simulink library "pdc_grc"  (R2024a)
settings: Solver=VariableStepAuto  StartTime=0.0  StopTime=10.0  RelTol=1e-3
undefined symbols (not defined in the file or in its folder): ENUM_IVTROPMODE_ASCHI, ENUM_IVTROPMODE_ASCLO, ENUM_IVTROPMODE_DTCYCTRL, ENUM_IVTROPMODE_FW, ENUM_IVTROPMODE_IVTROFF, KASC_DecDuty_value, KASC_OpenTime_s, KCCM_ASCSwitchEna_flg, KDSM_bIvtrTarHiDebug_flg, KDSM_DiagSpdH_rpm, KDSM_DiagSpdL_rpm, KeMCCR_b_UseMeasCrntDTC, KeSVMR_b_UseStrictClamp, KeSVMR_FullDTCCurr_A, KeSVMR_PWMPrd_cnt, KeSVMR_StrClampMaxDuty_pct, KeSVMR_StrClampMinDuty_pct, KeSVMR_t_DeadTime, KeSVMR_t_MinPulseWidth, KOSP_IvtrTarMor_enum_ovrdflg, KOSP_IvtrTarMor_enum_ovrdval, KPDC_facScalePWM_C, KPDC_FWCnt_C, KPDC_nPosnErrMaxSpd_C, StIvtrMod, StMotMod
libraries: simulink x18, GRC_Lib x6
(part 1 of 3)
settings Model: Creator=FVT22063  LastModifiedBy=FVT22063
settings SFSimCC: SimCustomHeaderCode="#include \"FVTMC_API.h\""  SimUserSources=FVTMC_API.c

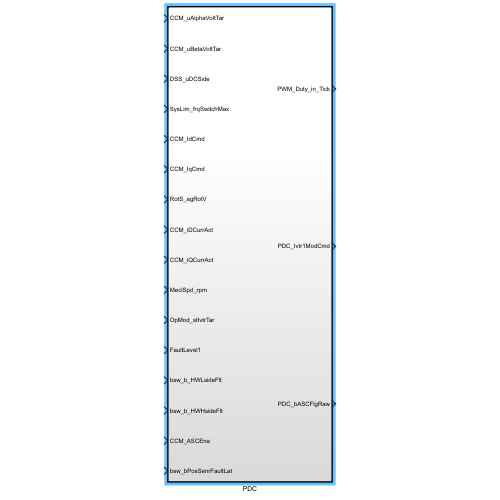
[thumbnail: Simulink's stored preview of the top-level diagram]
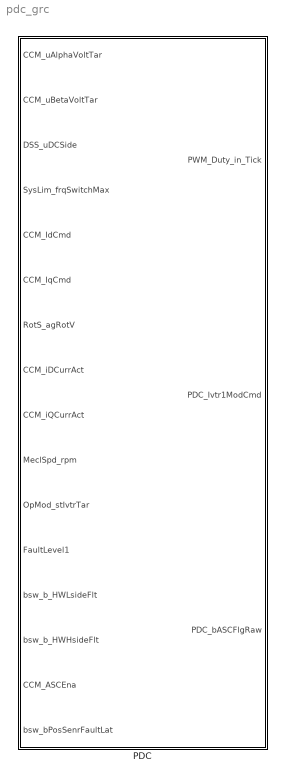
== system pdc_grc ==
  PDC : Subsystem  TreatAsAtomicUnit=on
      settings: RTWSystemCode=Nonreusable function  RTWFcnNameOpts=Use subsystem name  RTWFileNameOpts=Use subsystem name

== system pdc_grc/PDC ==
  CCM_uAlphaVoltTar : Inport  OutDataTypeStr=single
  CCM_uBetaVoltTar : Inport  Port=2  OutDataTypeStr=single
  DSS_uDCSide : Inport  Port=3  OutDataTypeStr=single
  SysLim_frqSwitchMax : Inport  Port=4  OutDataTypeStr=single
  CCM_IdCmd : Inport  Port=5  OutDataTypeStr=single
  CCM_IqCmd : Inport  Port=6  OutDataTypeStr=single
  RotS_agRotV : Inport  Port=7  OutDataTypeStr=single
  CCM_iDCurrAct : Inport  Port=8  OutDataTypeStr=single
  CCM_iQCurrAct : Inport  Port=9  OutDataTypeStr=single
  MeclSpd_rpm : Inport  Port=10  OutDataTypeStr=single
  OpMod_stIvtrTar : Inport  Port=11
  FaultLevel1 : Inport  Port=12  OutDataTypeStr=boolean
  bsw_b_HWLsideFlt : Inport  Port=13  OutDataTypeStr=boolean
  bsw_b_HWHsideFlt : Inport  Port=14  OutDataTypeStr=boolean
  CCM_ASCEna : Inport  Port=15
  bsw_bPosSenrFaultLat : Inport  Port=16  OutDataTypeStr=boolean
  Bus Creator : BusCreator  Inputs=4
  Bus Selector : BusSelector  OutputSignals=CCM_uAlphaVoltTar,CCM_uBetaVoltTar
  Bus Selector1 : BusSelector  OutputSignals=CCM_uAlphaVoltTar,CCM_uBetaVoltTar,DSS_uDCSide,SysLim_frqSwitchMax
  Bus Selector2 : BusSelector  OutputSignals=SysLim_frqSwitchMax
  ChangeTimeCalculation : Subsystem
  PWMCalculation : Subsystem
  SectorDetermine : Subsystem
  WorkTimeCalculation : Subsystem
  PWM_Duty_in_Tick : Outport  VectorParamsAs1DForOutWhenUnconnected=off
  PDC_Ivtr1ModCmd : Outport  Port=2  VectorParamsAs1DForOutWhenUnconnected=off
  PDC_bASCFlgRaw : Outport  Port=3  VectorParamsAs1DForOutWhenUnconnected=off
  wires:
  Bus Creator/1 -> Bus Selector1/1, Bus Selector2/1, Bus Selector/1
  Bus Selector1/1 -> WorkTimeCalculation/1(CCM_uAlphaVoltTar)  "<CCM_uAlphaVoltTar>"
  WorkTimeCalculation/1(PDC_tiWork1) -> ChangeTimeCalculation/1(PDC_tiWork1)
  Bus Selector2/1 -> PWMCalculation/2(SysLim_frqSwitchMax), ChangeTimeCalculation/4(SysLim_frqSwitchMax)  "<SysLim_frqSwitchMax>"
  Bus Selector1/3 -> WorkTimeCalculation/3(DSS_uDCSide)  "<DSS_uDCSide>"
  Bus Selector1/2 -> WorkTimeCalculation/2(CCM_uBetaVoltTar)  "<CCM_uBetaVoltTar>"
  ChangeTimeCalculation/1(PDC_tiChangeAry) -> PWMCalculation/1(PDC_tiChangeAry)
  Bus Selector/2 -> SectorDetermine/2(CCM_uBetaVoltTar)  "<CCM_uBetaVoltTar>"
  SectorDetermine/1(PDC_noSector) -> WorkTimeCalculation/5(PDC_noSector), ChangeTimeCalculation/3(PDC_noSector)
  Bus Selector1/4 -> WorkTimeCalculation/4(SysLim_frqSwitchMax)  "<SysLim_frqSwitchMax>"
  CCM_uAlphaVoltTar/1 -> Bus Creator/2  "CCM_uAlphaVoltTar"
  WorkTimeCalculation/2(PDC_tiWork2) -> ChangeTimeCalculation/2(PDC_tiWork2)
  Bus Selector/1 -> SectorDetermine/1(CCM_uAlphaVoltTar)  "<CCM_uAlphaVoltTar>"
  CCM_uBetaVoltTar/1 -> Bus Creator/3  "CCM_uBetaVoltTar"
  DSS_uDCSide/1 -> Bus Creator/1  "DSS_uDCSide"
  SysLim_frqSwitchMax/1 -> Bus Creator/4  "SysLim_frqSwitchMax"
  PWMCalculation/2(PDC_Ivtr1ModCmd) -> PDC_Ivtr1ModCmd/1
  CCM_IdCmd/1 -> PWMCalculation/3(CCM_IdCmd)
  CCM_IqCmd/1 -> PWMCalculation/4(CCM_IqCmd)
  RotS_agRotV/1 -> PWMCalculation/5(RotS_agRotV)
  CCM_iDCurrAct/1 -> PWMCalculation/6(CCM_iDCurrAct)
  CCM_iQCurrAct/1 -> PWMCalculation/7(CCM_iQCurrAct)
  PWMCalculation/3(PDC_bASCFlgRaw) -> PDC_bASCFlgRaw/1
  OpMod_stIvtrTar/1 -> PWMCalculation/9(OpMod_stIvtrTar)
  MeclSpd_rpm/1 -> PWMCalculation/8(MeclSpd_rpm)
  FaultLevel1/1 -> PWMCalculation/10(FaultLevel2)
  bsw_b_HWLsideFlt/1 -> PWMCalculation/11(bsw_b_HWLsideFlt)
  bsw_b_HWHsideFlt/1 -> PWMCalculation/12(bsw_b_HWHsideFlt)
  CCM_ASCEna/1 -> PWMCalculation/13(CCM_ASCEna)
  bsw_bPosSenrFaultLat/1 -> PWMCalculation/14(bsw_bPosSenrFaultLat)
  PWMCalculation/1(PWM_Duty_in_Tick) -> PWM_Duty_in_Tick/1

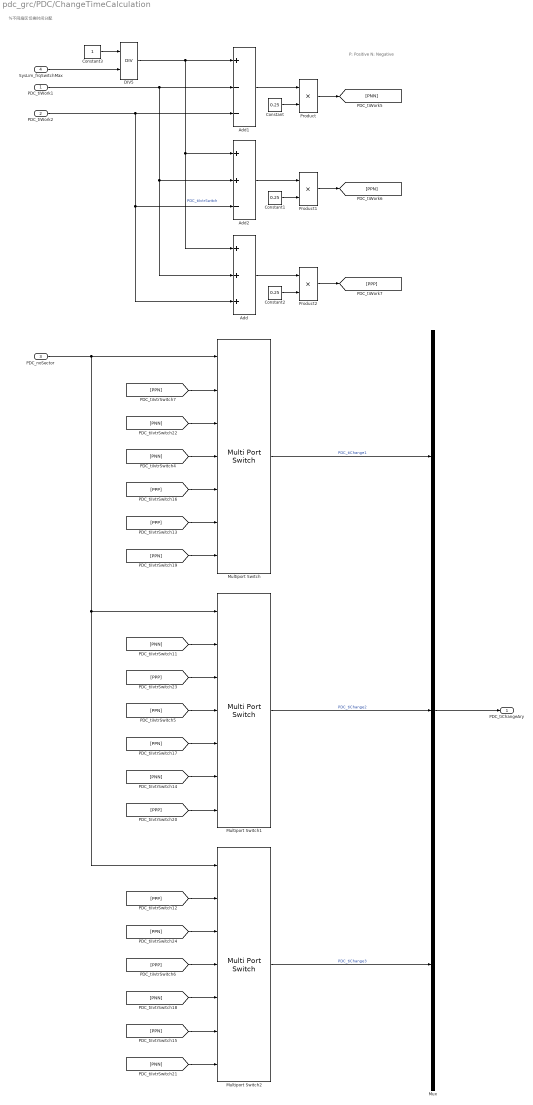
== system pdc_grc/PDC/ChangeTimeCalculation ==
  note: P: Positive
      | N: Negative
  note: %不同扇区切换时间分配
  PDC_tiWork1 : Inport  OutDataTypeStr=single
  PDC_tiWork2 : Inport  Port=2  OutDataTypeStr=single
  PDC_noSector : Inport  Port=3  OutDataTypeStr=single
  SysLim_frqSwitchMax : Inport  Port=4  OutDataTypeStr=single
  Add : Sum  Inputs=+++
  Add1 : Sum  Inputs=+--
  Add2 : Sum  Inputs=++-
  Constant : Constant  Value=0.25  OutDataTypeStr=single
  Constant1 : Constant  Value=0.25  OutDataTypeStr=single
  Constant2 : Constant  Value=0.25  OutDataTypeStr=single
  Constant3 : Constant  OutDataTypeStr=single
  DIV5 : GRC_Lib/ArithmeticOperations/DIV  MinDivVal=1e-15  IpDT=single
  Multiport Switch : MultiPortSwitch  Inputs=6  DiagnosticForDefault=None  SaturateOnIntegerOverflow=off  InputSameDT=off
  Multiport Switch1 : MultiPortSwitch  Inputs=6  DiagnosticForDefault=None  SaturateOnIntegerOverflow=off  InputSameDT=off
  Multiport Switch2 : MultiPortSwitch  Inputs=6  DiagnosticForDefault=None  SaturateOnIntegerOverflow=off  InputSameDT=off
  Mux : Mux  Inputs=3
  Product : Product
  Product1 : Product
  Product2 : Product
  PDC_tiChangeAry : Outport  OutDataTypeStr=single  VectorParamsAs1DForOutWhenUnconnected=off
  wires:
  DIV5/1 -> Add/1, Add2/1, Add1/1  "PDC_tiIvtrSwitch"
  PDC_tiWork1/1 -> Add/2, Add2/2, Add1/2
  PDC_tiWork2/1 -> Add1/3, Add/3, Add2/3
  PDC_noSector/1 -> Multiport Switch2/1, Multiport Switch1/1, Multiport Switch/1
  Add1/1 -> Product/1
  Product/1 -> [PNN]
  Constant/1 -> Product/2
  Constant1/1 -> Product1/2
  Product1/1 -> [PPN]
  Add2/1 -> Product1/1
  Add/1 -> Product2/1
  Product2/1 -> [PPP]
  Constant2/1 -> Product2/2
  Multiport Switch/1 -> Mux/1  "PDC_tiChange1"
  Multiport Switch1/1 -> Mux/2  "PDC_tiChange2"
  Multiport Switch2/1 -> Mux/3  "PDC_tiChange3"
  [PNN] -> Multiport Switch/4
  [PPN] -> Multiport Switch1/4
  [PPP] -> Multiport Switch2/4
  [PPN] -> Multiport Switch/2
  [PNN] -> Multiport Switch1/2
  [PPP] -> Multiport Switch2/2
  [PPP] -> Multiport Switch/6
  [PNN] -> Multiport Switch1/6
  [PPN] -> Multiport Switch2/6
  [PPP] -> Multiport Switch/5
  [PPN] -> Multiport Switch1/5
  [PNN] -> Multiport Switch2/5
  [PPN] -> Multiport Switch/7
  [PPP] -> Multiport Switch1/7
  [PNN] -> Multiport Switch2/7
  [PNN] -> Multiport Switch/3
  [PPP] -> Multiport Switch1/3
  [PPN] -> Multiport Switch2/3
  SysLim_frqSwitchMax/1 -> DIV5/2
  Constant3/1 -> DIV5/1
  Mux/1 -> PDC_tiChangeAry/1

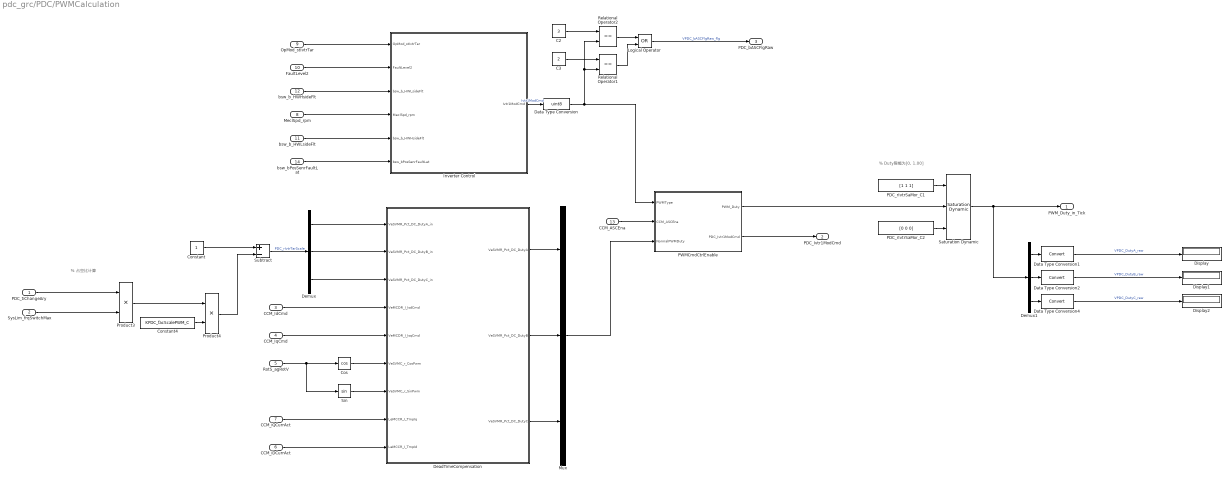
== system pdc_grc/PDC/PWMCalculation ==
  note: % 占空比计算
  note: % Duty限幅为[0, 1.00]
  PDC_tiChangeAry : Inport
  SysLim_frqSwitchMax : Inport  Port=2  OutDataTypeStr=single
  CCM_IdCmd : Inport  Port=3  OutDataTypeStr=single
  CCM_IqCmd : Inport  Port=4  OutDataTypeStr=single
  RotS_agRotV : Inport  Port=5  OutDataTypeStr=single
  CCM_iDCurrAct : Inport  Port=6  OutDataTypeStr=single
  CCM_iQCurrAct : Inport  Port=7  OutDataTypeStr=single
  MeclSpd_rpm : Inport  Port=8  OutDataTypeStr=single
  OpMod_stIvtrTar : Inport  Port=9
  FaultLevel2 : Inport  Port=10  OutDataTypeStr=boolean
  bsw_b_HWLsideFlt : Inport  Port=11
  bsw_b_HWHsideFlt : Inport  Port=12
  CCM_ASCEna : Inport  Port=13
  bsw_bPosSenrFaultLat : Inport  Port=14  OutDataTypeStr=boolean
  C2 : Constant  Value=3  OutDataTypeStr=uint8  SampleTime=-1
  C3 : Constant  Value=2  OutDataTypeStr=uint8  SampleTime=-1
  Constant : Constant  OutDataTypeStr=Inherit: Inherit via back propagation
  Constant4 : Constant  Value=KPDC_facScalePWM_C
  Cos : Trigonometry  Operator=cos
  Data Type Conversion : DataTypeConversion  OutDataTypeStr=uint8  SaturateOnIntegerOverflow=off  RndMeth=Floor
  Data Type Conversion1 : DataTypeConversion  SaturateOnIntegerOverflow=off  RndMeth=Floor
  Data Type Conversion2 : DataTypeConversion  SaturateOnIntegerOverflow=off  RndMeth=Floor
  Data Type Conversion4 : DataTypeConversion  SaturateOnIntegerOverflow=off  RndMeth=Floor
  DeadTimeCompensation : Subsystem
  Demux : Demux  Outputs=3
  Demux1 : Demux  Outputs=3
  Display : Display
  Display1 : Display
  Display2 : Display
  "Inverter Control " : Subsystem
  Logical Operator : Logic  Operator=OR  AllPortsSameDT=off  OutDataTypeStr=boolean
  Mux : Mux  Inputs=3
  PDC_rIvtrSaMor_C1 : Constant  Value=[1 1 1]
  PDC_rIvtrSaMor_C2 : Constant  Value=[0 0 0]
  PWMCmdCtrlEnable : Subsystem
      settings: FunctionInterfaceSpec=Allow arguments (Optimized)
  Product3 : Product
  Product4 : Product
  Relational Operator1 : RelationalOperator  Operator===  OutDataTypeStr=boolean  RndMeth=Simplest  InputSameDT=off
  Relational Operator2 : RelationalOperator  Operator===  OutDataTypeStr=boolean  RndMeth=Simplest  InputSameDT=off
  Saturation Dynamic : simulink/Discontinuities/Saturation Dynamic  OutMin=[]  OutMax=[]  OutDataTypeStr=Inherit: Same as second input  OutDataType=fixdt(1, 16)  OutScaling=2^-10  DoSatur=off
  Sin : Trigonometry
  Subtract : Sum  Inputs=+-
  PWM_Duty_in_Tick : Outport
  PDC_Ivtr1ModCmd : Outport  Port=2  OutDataTypeStr=uint8  VectorParamsAs1DForOutWhenUnconnected=off
  PDC_bASCFlgRaw : Outport  Port=3  VectorParamsAs1DForOutWhenUnconnected=off
  wires:
  Product4/1 -> Subtract/2
  PDC_rIvtrSaMor_C2/1 -> Saturation Dynamic/3
  PDC_rIvtrSaMor_C1/1 -> Saturation Dynamic/1
  Constant4/1 -> Product4/2
  Product3/1 -> Product4/1
  SysLim_frqSwitchMax/1 -> Product3/2
  PDC_tiChangeAry/1 -> Product3/1
  Saturation Dynamic/1 -> Demux1/1, PWM_Duty_in_Tick/1
  Cos/1 -> DeadTimeCompensation/6(VeSVMC_r_CosPwm)
  CCM_IdCmd/1 -> DeadTimeCompensation/4(VeMCDR_I_IsdCmd)
  Demux/1 -> DeadTimeCompensation/1(VeSVMR_Pct_DC_DutyA_in)
  Sin/1 -> DeadTimeCompensation/7(VeSVMC_r_SinPwm)
  Demux/2 -> DeadTimeCompensation/2(VeSVMR_Pct_DC_DutyB_in)
  CCM_IqCmd/1 -> DeadTimeCompensation/5(VeMCDR_I_IsqCmd)
  Demux/3 -> DeadTimeCompensation/3(VeSVMR_Pct_DC_DutyC_in)
  RotS_agRotV/1 -> Sin/1, Cos/1
  DeadTimeCompensation/1(VeSVMR_Pct_DC_DutyA) -> Mux/1
  DeadTimeCompensation/2(VeSVMR_Pct_DC_DutyB) -> Mux/2
  DeadTimeCompensation/3(VeSVMR_Pct_DC_DutyC) -> Mux/3
  PWMCmdCtrlEnable/1(PWM_Duty) -> Saturation Dynamic/2
  Constant/1 -> Subtract/1
  Subtract/1 -> Demux/1  "PDC_rIvtrTarScale"
  PWMCmdCtrlEnable/2(PDC_Ivtr1ModCmd) -> PDC_Ivtr1ModCmd/1
  Mux/1 -> PWMCmdCtrlEnable/3(NormalPWMDuty)
  CCM_iQCurrAct/1 -> DeadTimeCompensation/8(LeMCCR_I_TmpIq)
  CCM_iDCurrAct/1 -> DeadTimeCompensation/9(LeMCCR_I_TmpId)
  OpMod_stIvtrTar/1 -> "Inverter Control "/1(OpMod_stIvtrTar)
  MeclSpd_rpm/1 -> "Inverter Control "/4(MeclSpd_rpm)
  "Inverter Control "/1(Ivtr1ModCmd) -> Data Type Conversion/1  "Ivtr1ModCmd"
  bsw_b_HWLsideFlt/1 -> "Inverter Control "/5(bsw_b_HWHsideFlt)
  FaultLevel2/1 -> "Inverter Control "/2(FaultLevel2)
  bsw_b_HWHsideFlt/1 -> "Inverter Control "/3(bsw_b_HWLsideFlt)
  Data Type Conversion/1 -> Relational Operator2/2, Relational Operator1/2, PWMCmdCtrlEnable/1(PWMType)
  CCM_ASCEna/1 -> PWMCmdCtrlEnable/2(CCM_ASCEna)
  C2/1 -> Relational Operator2/1
  C3/1 -> Relational Operator1/1
  Relational Operator2/1 -> Logical Operator/1
  Relational Operator1/1 -> Logical Operator/2
  Logical Operator/1 -> PDC_bASCFlgRaw/1  "VPDC_bASCFlgRaw_flg"
  bsw_bPosSenrFaultLat/1 -> "Inverter Control "/6(bsw_bPosSenrFaultLat)
  Demux1/1 -> Data Type Conversion1/1
  Demux1/2 -> Data Type Conversion2/1
  Demux1/3 -> Data Type Conversion4/1
  Data Type Conversion1/1 -> Display/1  "VPDC_DutyA_raw"
  Data Type Conversion2/1 -> Display1/1  "VPDC_DutyB_raw"
  Data Type Conversion4/1 -> Display2/1  "VPDC_DutyC_raw"

== system pdc_grc/PDC/SectorDetermine ==
  note: 扇区
      | Ⅰ
      | Ⅱ
      | Ⅲ
      | Ⅳ
      | Ⅴ
      | Ⅵ
      |
      | N
      | 3
      | 1
      | 5
      | 4
      | 6
      | 2
  note: C
  note: B
  note: A
  note: %扇区判断
  CCM_uAlphaVoltTar : Inport  OutDataTypeStr=single
  CCM_uBetaVoltTar : Inport  Port=2  OutDataTypeStr=single
  Add : Sum  Inputs=3
  Constant : Constant  Value=0.866  OutDataTypeStr=single
  Constant1 : Constant  Value=0.5  OutDataTypeStr=single
  Constant2 : Constant  Value=-1  OutDataTypeStr=single
  Constant3 : Constant  Value=0  OutDataTypeStr=single
  Constant4 : Constant  Value=2  OutDataTypeStr=single
  Constant5 : Constant  Value=4  OutDataTypeStr=single
  Constant6 : Constant  OutDataTypeStr=single
  Product{,1..5} (6 alike) : Product
  Relational Operator : RelationalOperator  OutDataTypeStr=boolean  RndMeth=Simplest  InputSameDT=off
  Relational Operator1 : RelationalOperator  OutDataTypeStr=boolean  RndMeth=Simplest  InputSameDT=off
  Relational Operator2 : RelationalOperator  OutDataTypeStr=boolean  RndMeth=Simplest  InputSameDT=off
  PDC_noSector : Outport  OutDataTypeStr=single  VectorParamsAs1DForOutWhenUnconnected=off
  wires:
  CCM_uAlphaVoltTar/1 -> Product/1  "CCM_uAlphaVoltTar"
  Constant/1 -> Product/2
  CCM_uBetaVoltTar/1 -> Relational Operator2/1, Product1/1  "CCM_uBetaVoltTar"
  Constant1/1 -> Product1/2
  Product/1 -> Product2/1, Relational Operator/1
  Product1/1 -> Relational Operator/2, Relational Operator1/2
  Product2/1 -> Relational Operator1/1
  Constant2/1 -> Product2/2
  Constant3/1 -> Relational Operator2/2
  Relational Operator/1 -> Product3/1
  Constant4/1 -> Product3/2
  Constant5/1 -> Product4/2
  Relational Operator1/1 -> Product4/1
  Constant6/1 -> Product5/2
  Relational Operator2/1 -> Product5/1
  Product3/1 -> Add/1
  Product4/1 -> Add/2
  Product5/1 -> Add/3
  Add/1 -> PDC_noSector/1  "PDC_noSector"

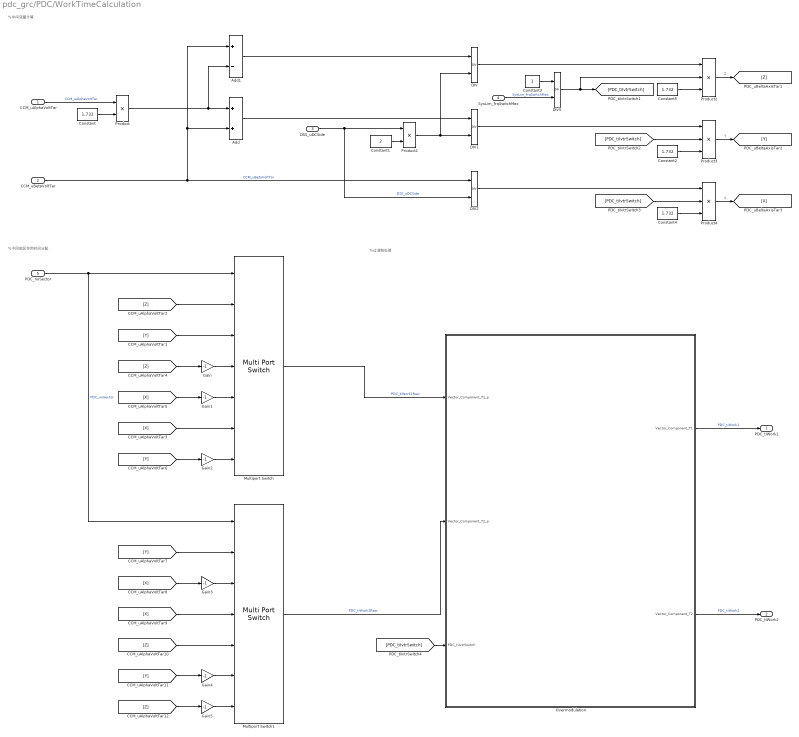
== system pdc_grc/PDC/WorkTimeCalculation ==
  note: %过调制处理
  note: %中间变量计算
  note: %不同扇区作用时间分配
  CCM_uAlphaVoltTar : Inport  OutDataTypeStr=single
  CCM_uBetaVoltTar : Inport  Port=2  OutDataTypeStr=single
  DSS_uDCSide : Inport  Port=3  OutDataTypeStr=single
  SysLim_frqSwitchMax : Inport  Port=4  OutDataTypeStr=single
  PDC_noSector : Inport  Port=5  OutDataTypeStr=single
  Add : Sum
  Add1 : Sum  Inputs=+-
  Constant{,2,4..5} (4 alike) : Constant  Value=1.732  OutDataTypeStr=single
  Constant1 : Constant  Value=2  OutDataTypeStr=single
  Constant3 : Constant  OutDataTypeStr=single
  DIV{,1..2,5} (4 alike) : GRC_Lib/ArithmeticOperations/DIV  MinDivVal=1e-15  IpDT=single
  Gain{,1..5} (6 alike) : Gain  Gain=-1
  Multiport Switch : MultiPortSwitch  Inputs=6  DiagnosticForDefault=None  SaturateOnIntegerOverflow=off  InputSameDT=off
  Multiport Switch1 : MultiPortSwitch  Inputs=6  DiagnosticForDefault=None  SaturateOnIntegerOverflow=off  InputSameDT=off
  Overmodulation : Subsystem
  Product : Product
  Product1 : Product
  Product2 : Product  Inputs=3
  Product3 : Product  Inputs=3
  Product4 : Product  Inputs=3
  PDC_tiWork1 : Outport  OutDataTypeStr=single  VectorParamsAs1DForOutWhenUnconnected=off
  PDC_tiWork2 : Outport  Port=2  OutDataTypeStr=single  VectorParamsAs1DForOutWhenUnconnected=off
  wires:
  Constant/1 -> Product/2
  CCM_uAlphaVoltTar/1 -> Product/1  "CCM_uAlphaVoltTar"
  Product/1 -> Add1/2, Add/1
  Add1/1 -> DIV/1
  Constant1/1 -> Product1/2
  DIV/1 -> Product2/1
  Constant5/1 -> Product2/3
  DIV5/1 -> [PDC_tiIvtrSwitch], Product2/2
  Product2/1 -> [Z]  "Z"
  Product3/1 -> [Y]  "Y"
  Constant2/1 -> Product3/3
  DIV1/1 -> Product3/1
  Product1/1 -> DIV/2, DIV1/2
  DSS_uDCSide/1 -> DIV2/2, Product1/1  "DSS_uDCSide"
  Add/1 -> DIV1/1
  CCM_uBetaVoltTar/1 -> Add1/1, Add/2, DIV2/1  "CCM_uBetaVoltTar"
  DIV2/1 -> Product4/1
  Constant4/1 -> Product4/3
  Product4/1 -> [X]  "X"
  PDC_noSector/1 -> Multiport Switch1/1, Multiport Switch/1  "PDC_noSector"
  [Z] -> Multiport Switch/2
  [Y] -> Multiport Switch/3
  [Z] -> Gain/1
  Gain/1 -> Multiport Switch/4
  [X] -> Multiport Switch/6
  [X] -> Gain1/1
  Gain1/1 -> Multiport Switch/5
  [Y] -> Gain2/1
  Gain2/1 -> Multiport Switch/7
  [Y] -> Multiport Switch1/2
  Gain3/1 -> Multiport Switch1/3
  [X] -> Gain3/1
  [X] -> Multiport Switch1/4
  [Z] -> Multiport Switch1/5
  Gain4/1 -> Multiport Switch1/6
  [Y] -> Gain4/1
  Gain5/1 -> Multiport Switch1/7
  [Z] -> Gain5/1
  Overmodulation/1(Vector_Component_T1) -> PDC_tiWork1/1  "PDC_tiWork1"
  Overmodulation/2(Vector_Component_T2) -> PDC_tiWork2/1  "PDC_tiWork2"
  [PDC_tiIvtrSwitch] -> Product3/2
  [PDC_tiIvtrSwitch] -> Product4/2
  SysLim_frqSwitchMax/1 -> DIV5/2  "SysLim_frqSwitchMax"
  Constant3/1 -> DIV5/1
  Multiport Switch/1 -> Overmodulation/1(Vector_Component_T1_p)  "PDC_tiWork1Raw"
  Multiport Switch1/1 -> Overmodulation/2(Vector_Component_T2_p)  "PDC_tiWork2Raw"
  [PDC_tiIvtrSwitch] -> Overmodulation/3(PDC_tiIvtrSwitch)

== system pdc_grc/PDC/PWMCalculation/DeadTimeCompensation ==
  VeSVMR_Pct_DC_DutyA_in : Inport
  VeSVMR_Pct_DC_DutyB_in : Inport  Port=2
  VeSVMR_Pct_DC_DutyC_in : Inport  Port=3
  VeMCDR_I_IsdCmd : Inport  Port=4
  VeMCDR_I_IsqCmd : Inport  Port=5
  VeSVMC_r_CosPwm : Inport  Port=6
  VeSVMC_r_SinPwm : Inport  Port=7
  LeMCCR_I_TmpIq : Inport  Port=8
  LeMCCR_I_TmpId : Inport  Port=9
  MngSVMR_Base_MtrCntrl0_ProcessDCsForHWIO : Subsystem  RTWFcnName=MngSVMR_Base_MtrCntrl0_ProcessDCsForHWIO  RTWFileName=svmcmbas
      settings: RTWSystemCode=Nonreusable function  RTWFcnNameOpts=User specified  RTWFileNameOpts=User specified
  ReInitSVMR_DeadTimeCompensation : Subsystem  TreatAsAtomicUnit=on  RTWFcnName=ReInitSVMR_DeadTimeCompensation  RTWFileName=svmcmbas
      settings: RTWFcnNameOpts=User specified  RTWFileNameOpts=User specified
  ReInitSVMR_PWM_Modulation : Subsystem  TreatAsAtomicUnit=on  RTWFcnName=ReInitSVMR_PWM_Modulation  RTWFileName=svmcmbas
      settings: RTWFcnNameOpts=User specified  RTWFileNameOpts=User specified
  ReciSqrt3M1 : Constant  Value=KeMCCR_b_UseMeasCrntDTC  OutDataTypeStr=uint8
      settings: AttributesFormatString=dd_value = 0
  ReciSqrt3M2 : Constant  OutDataTypeStr=uint8
      settings: AttributesFormatString=dd_value = 1
  ReciSqrt3M3 : Constant  OutDataTypeStr=uint8
      settings: AttributesFormatString=dd_value = 1
  Terminator : Terminator
  Terminator1 : Terminator
  Terminator2 : Terminator
  VeSVMR_Pct_DC_DutyA : Outport  VectorParamsAs1DForOutWhenUnconnected=off
  VeSVMR_Pct_DC_DutyB : Outport  Port=2  VectorParamsAs1DForOutWhenUnconnected=off
  VeSVMR_Pct_DC_DutyC : Outport  Port=3  VectorParamsAs1DForOutWhenUnconnected=off
  wires:
  MngSVMR_Base_MtrCntrl0_ProcessDCsForHWIO/4(VeSVMR_Pct_DC_DutyA) -> VeSVMR_Pct_DC_DutyA/1
  MngSVMR_Base_MtrCntrl0_ProcessDCsForHWIO/5(VeSVMR_Pct_DC_DutyB) -> VeSVMR_Pct_DC_DutyB/1
  VeSVMR_Pct_DC_DutyB_in/1 -> MngSVMR_Base_MtrCntrl0_ProcessDCsForHWIO/3(VeSVMR_Pct_DC_DutyB_in)
  MngSVMR_Base_MtrCntrl0_ProcessDCsForHWIO/1(VeSVMR_Pct_DC_DutyA_Cmd) -> Terminator/1
  MngSVMR_Base_MtrCntrl0_ProcessDCsForHWIO/6(VeSVMR_Pct_DC_DutyC) -> VeSVMR_Pct_DC_DutyC/1
  MngSVMR_Base_MtrCntrl0_ProcessDCsForHWIO/2(VeSVMR_Pct_DC_DutyB_Cmd) -> Terminator1/1
  VeSVMR_Pct_DC_DutyA_in/1 -> MngSVMR_Base_MtrCntrl0_ProcessDCsForHWIO/2(VeSVMR_Pct_DC_DutyA_in)
  ReciSqrt3M3/1 -> MngSVMR_Base_MtrCntrl0_ProcessDCsForHWIO/1(VeGDCR_e_EffectivePwrStageCmd)
  MngSVMR_Base_MtrCntrl0_ProcessDCsForHWIO/3(VeSVMR_Pct_DC_DutyC_Cmd) -> Terminator2/1
  VeMCDR_I_IsqCmd/1 -> MngSVMR_Base_MtrCntrl0_ProcessDCsForHWIO/6(VeMCDR_I_IsqCmd)
  VeSVMR_Pct_DC_DutyC_in/1 -> MngSVMR_Base_MtrCntrl0_ProcessDCsForHWIO/4(VeSVMR_Pct_DC_DutyC_in)
  VeMCDR_I_IsdCmd/1 -> MngSVMR_Base_MtrCntrl0_ProcessDCsForHWIO/5(VeMCDR_I_IsdCmd)
  VeSVMC_r_CosPwm/1 -> MngSVMR_Base_MtrCntrl0_ProcessDCsForHWIO/7(VeSVMC_r_CosPwm)
  VeSVMC_r_SinPwm/1 -> MngSVMR_Base_MtrCntrl0_ProcessDCsForHWIO/8(VeSVMC_r_SinPwm)
  LeMCCR_I_TmpIq/1 -> MngSVMR_Base_MtrCntrl0_ProcessDCsForHWIO/18(LeMCCR_I_TmpIq)
  LeMCCR_I_TmpId/1 -> MngSVMR_Base_MtrCntrl0_ProcessDCsForHWIO/19(LeMCCR_I_TmpId)
  ReciSqrt3M2/1 -> MngSVMR_Base_MtrCntrl0_ProcessDCsForHWIO/11(VeSVMR_e_PWM_Type)
  ReInitSVMR_DeadTimeCompensation/1(VeSVMR_K_DeadTimeCmp_Slope) -> MngSVMR_Base_MtrCntrl0_ProcessDCsForHWIO/9(VaSVMR_K_DeadTimeCmp_Slope)
  ReInitSVMR_DeadTimeCompensation/2(VeSVMR_Pct_DeadTimeCmp) -> MngSVMR_Base_MtrCntrl0_ProcessDCsForHWIO/10(VaSVMR_Pct_DeadTimeCmp)
  ReInitSVMR_PWM_Modulation/1(VeSVMR_Pct_DC_FixedDutyOffset) -> MngSVMR_Base_MtrCntrl0_ProcessDCsForHWIO/12(VeSVMR_Pct_DC_FixedDutyOffset)
  ReInitSVMR_PWM_Modulation/2(VeSVMR_Pct_DCMaxDuty_nom) -> MngSVMR_Base_MtrCntrl0_ProcessDCsForHWIO/13(VaSVMR_Pct_DCMaxDuty_nom)
  ReInitSVMR_PWM_Modulation/3(VeSVMR_Pct_DCMinDuty_nom) -> MngSVMR_Base_MtrCntrl0_ProcessDCsForHWIO/14(VaSVMR_Pct_DCMinDuty_nom)
  ReInitSVMR_PWM_Modulation/4(VeSVMR_Pct_DCMaxDutyRound) -> MngSVMR_Base_MtrCntrl0_ProcessDCsForHWIO/15(VaSVMR_Pct_DCMaxDutyRound)
  ReInitSVMR_PWM_Modulation/5(VeSVMR_Pct_DCMinDutyRound) -> MngSVMR_Base_MtrCntrl0_ProcessDCsForHWIO/16(VaSVMR_Pct_DCMinDutyRound)
  ReciSqrt3M1/1 -> MngSVMR_Base_MtrCntrl0_ProcessDCsForHWIO/17(VeMCCR_b_UseMeasCrntDTC)

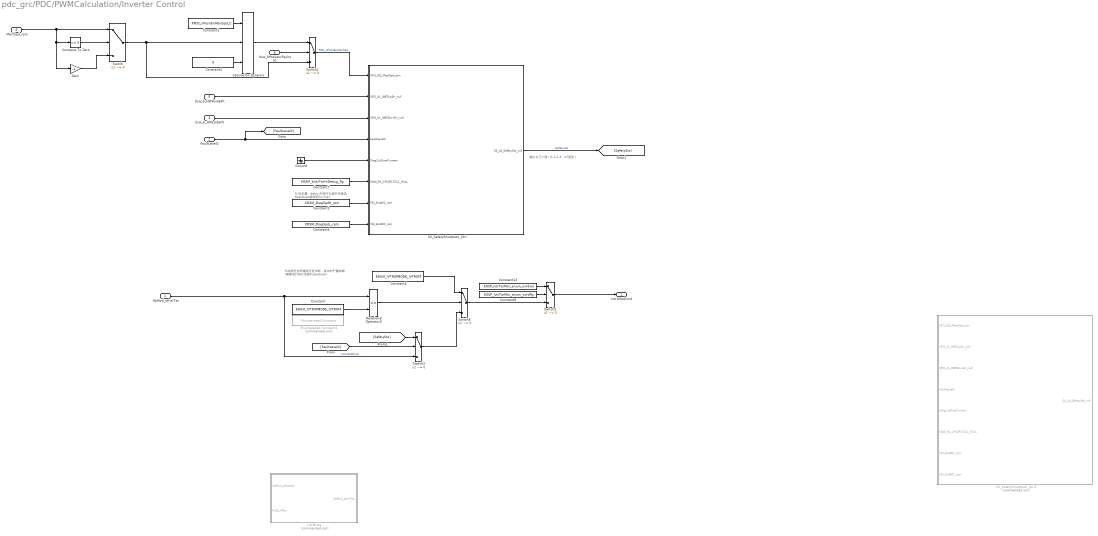
== system pdc_grc/PDC/PWMCalculation/Inverter Control  ==
  note: % 标定量，debug时候可以使开关管由
      | freewheel跳转到normal
  note: 输出为几个值（0-1-2-3，u8类型）
  note: %快速任务和慢速任务诊断，其中的严重故障
      | (需要进行ASC或者Freewheel)
  OpMod_stIvtrTar : Inport
  FaultLevel2 : Inport  Port=2  OutDataTypeStr=boolean
  bsw_b_HWLsideFlt : Inport  Port=3
  MeclSpd_rpm : Inport  Port=4  OutDataTypeStr=single
  bsw_b_HWHsideFlt : Inport  Port=5
  bsw_bPosSenrFaultLat : Inport  Port=6  OutDataTypeStr=boolean
  Compare To Zero : simulink/Logic and Bit Operations/Compare To Zero  relop=>=  OutDataTypeStr=boolean
  Constant : Constant  Value=ENUM_IVTROPMODE_IVTROFF
  Constant1 : Constant  Value=KPDC_nPosnErrMaxSpd_C
  Constant12 : Constant  Value=KOSP_IvtrTarMor_enum_ovrdval  SampleTime=-1
  Constant2 : Constant  Value=KDSM_DiagSpdH_rpm  SampleTime=-1
  Constant3 : Constant  Value=0  OutDataTypeStr=single
  Constant4 : Constant  Value=KDSM_DiagSpdL_rpm  SampleTime=-1
  Constant5 : Constant  Value=ENUM_IVTROPMODE_IVTROFF
  Constant7 : Constant  Value=KDSM_bIvtrTarHiDebug_flg  OutDataTypeStr=boolean  SampleTime=-1
  Constant9 : Constant  Value=KOSP_IvtrTarMor_enum_ovrdflg  OutDataTypeStr=boolean  SampleTime=-1
  Enumerated Constant1 : simulink/Sources/Enumerated Constant  Commented=on  OutDataTypeStr=Enum: StIvtrMod  Value=StIvtrMod.StIvtrModIvtrOffMod  SampleTime=inf
  Gain : Gain  Gain=-1  OutDataTypeStr=single
  Ground : Ground
  IvtrMode : Subsystem  Commented=on
  Relational Operator2 : RelationalOperator  Operator===  OutDataTypeStr=boolean  RndMeth=Simplest  InputSameDT=off
  SS_SafetyShutdown_Ctrl : Stateflow chart  TreatAsAtomicUnit=on
  SS_SafetyShutdown_Ctrl1 : Stateflow chart  Commented=on  TreatAsAtomicUnit=on
  Saturation Dynamic : simulink/Discontinuities/Saturation Dynamic  OutMin=[]  OutMax=[]  OutDataTypeStr=Inherit: Same as second input  OutDataType=fixdt(1, 16)  OutScaling=2^-10  DoSatur=off
  Switch{,1..3,5} (5 alike) : Switch  Criteria=u2 ~= 0  SaturateOnIntegerOverflow=off  InputSameDT=off
  Ivtr1ModCmd : Outport
  wires:
  Switch5/1 -> Switch2/3
  bsw_b_HWLsideFlt/1 -> SS_SafetyShutdown_Ctrl/3(SPI2_b1_IGBTDwnErr_null)
  FaultLevel2/1 -> [FaultLevel2], SS_SafetyShutdown_Ctrl/4(FaultLevel2)
  Constant12/1 -> Switch2/1
  Switch2/1 -> Ivtr1ModCmd/1
  Constant9/1 -> Switch2/2
  Gain/1 -> Switch/3
  Constant7/1 -> SS_SafetyShutdown_Ctrl/6(DIAG_B1_CPLDFLTCLC_NULL)
  MeclSpd_rpm/1 -> Switch/1, Compare To Zero/1, Gain/1
  Compare To Zero/1 -> Switch/2
  SS_SafetyShutdown_Ctrl/1(SS_u8_SafetySts_null) -> [SafetySts]  "SafetySts"
  bsw_b_HWHsideFlt/1 -> SS_SafetyShutdown_Ctrl/2(SPI2_b1_IGBTUpErr_null)
  Ground/1 -> SS_SafetyShutdown_Ctrl/5(Diag1_bOverCurrent)
  Constant/1 -> Relational Operator2/2
  Relational Operator2/1 -> Switch5/2
  Constant5/1 -> Switch5/1
  Switch3/1 -> Switch5/3
  [FaultLevel2] -> Switch3/2
  [SafetySts] -> Switch3/1
  Constant4/1 -> SS_SafetyShutdown_Ctrl/8(f32_ExtASC_rpm)
  Constant2/1 -> SS_SafetyShutdown_Ctrl/7(f32_EntASC_rpm)
  OpMod_stIvtrTar/1 -> Relational Operator2/1, Switch3/3  "Ivtr1ModCmd"
  Constant1/1 -> Saturation Dynamic/1
  Saturation Dynamic/1 -> Switch1/1
  Switch/1 -> Switch1/3, Saturation Dynamic/2
  Constant3/1 -> Saturation Dynamic/3
  bsw_bPosSenrFaultLat/1 -> Switch1/2
  Switch1/1 -> SS_SafetyShutdown_Ctrl/1(SPI1_f32_MeclSpd_rpm)  "PDC_nPosnErrMaxSpd"

== system pdc_grc/PDC/PWMCalculation/PWMCmdCtrlEnable ==
  PWMType : Inport
  CCM_ASCEna : Inport  Port=2
  NormalPWMDuty : Inport  Port=3
  C1 : Constant  OutDataTypeStr=uint8  SampleTime=-1
  C2 : Constant  Value=2  OutDataTypeStr=uint8  SampleTime=-1
  C3 : Constant  Value=3  OutDataTypeStr=uint8  SampleTime=-1
  C4 : Constant  Value=0  OutDataTypeStr=uint8  SampleTime=-1
  If : If  NumInputs=5  IfExpression=u1==u2  ElseIfExpressions=(u1==u3|u1==u4),u1==u5
  Merge : Merge  Inputs=4
  Merge2 : Merge  Inputs=4
  NormalPWM : Subsystem  TreatAsAtomicUnit=on
      settings: RTWFcnNameOpts=Use subsystem name
  PWMFW : Subsystem  TreatAsAtomicUnit=on
      settings: RTWFcnNameOpts=Use subsystem name
  PWMGOFF : Subsystem  TreatAsAtomicUnit=on
      settings: RTWFcnNameOpts=Use subsystem name
  ThreePhaseSC : Subsystem  TreatAsAtomicUnit=on
      settings: RTWFcnNameOpts=Use subsystem name
  ThreePhaseSC1 : Subsystem  Commented=on  TreatAsAtomicUnit=on
      settings: RTWFcnNameOpts=Use subsystem name
  PWM_Duty : Outport  VectorParamsAs1DForOutWhenUnconnected=off
  PDC_Ivtr1ModCmd : Outport  Port=2  VectorParamsAs1DForOutWhenUnconnected=off
  wires:
  If/1 -> NormalPWM/Action
  NormalPWM/1(PWM_Duty) -> Merge/1
  Merge/1 -> PWM_Duty/1
  If/3 -> PWMFW/Action
  PWMType/1 -> [PWMType], If/1
  C1/1 -> If/2
  If/2 -> ThreePhaseSC/Action
  ThreePhaseSC/1(PWM_Duty) -> Merge/2
  PWMFW/1(PWM_Duty) -> Merge/3
  NormalPWM/2(PDC_Ivtr1ModCmd) -> Merge2/1
  ThreePhaseSC/2(PDC_Ivtr1ModCmd) -> Merge2/2
  PWMFW/2(PDC_Ivtr1ModCmd) -> Merge2/3
  C4/1 -> If/5
  [PWMType] -> ThreePhaseSC/2(PWMType)
  If/4 -> PWMGOFF/Action
  [PWMType] -> PWMGOFF/1(PWMType)
  PWMGOFF/1(PWM_Duty) -> Merge/4
  PWMGOFF/2(PDC_Ivtr1ModCmd) -> Merge2/4
  NormalPWMDuty/1 -> ThreePhaseSC/1(NormalPWMDuty), NormalPWM/1(Normal_PWM_Duty)
  C2/1 -> If/3
  C3/1 -> If/4
  CCM_ASCEna/1 -> ThreePhaseSC/3(CCM_ASCEna)
  Merge2/1 -> PDC_Ivtr1ModCmd/1  "VPDC_Ivtr1ModCmd_enum"

== system pdc_grc/PDC/WorkTimeCalculation/Overmodulation ==
  Vector_Component_T1_p : Inport  OutDataTypeStr=single
  Vector_Component_T2_p : Inport  Port=2  OutDataTypeStr=single
  PDC_tiIvtrSwitch : Inport  Port=3  OutDataTypeStr=single
  Overmodulation : Stateflow chart  Description=|  TreatAsAtomicUnit=on
      | The duty limitation, which limit to peak duty.
      | T1 = T1 * Duty_max / ( T1 + T2 );             
      | T2 = T2 * Duty_max / ( T1 + T2 );
  Vector_Component_T1 : Outport  OutDataTypeStr=single
  Vector_Component_T2 : Outport  Port=2  OutDataTypeStr=single
  wires:
  Overmodulation/2(TM_Vector_Component_T2) -> Vector_Component_T2/1
  Overmodulation/1(TM_Vector_Component_T1) -> Vector_Component_T1/1
  PDC_tiIvtrSwitch/1 -> Overmodulation/1(Duty_Max)
  Vector_Component_T1_p/1 -> Overmodulation/2(TM_Vector_Component_T1_p)
  Vector_Component_T2_p/1 -> Overmodulation/3(TM_Vector_Component_T2_p)

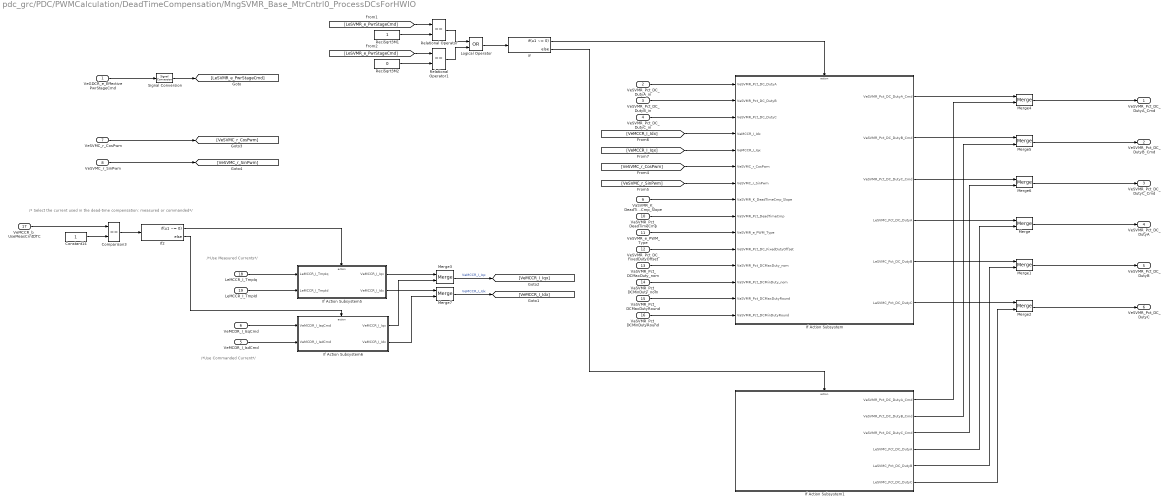
== system pdc_grc/PDC/PWMCalculation/DeadTimeCompensation/MngSVMR_Base_MtrCntrl0_ProcessDCsForHWIO ==
  note: /*Use Commanded Current*/
  note: /*Use Measured Currents*/
  note: /* Select the current used in the dead-time compensation: measured or commanded*/
  VeGDCR_e_EffectivePwrStageCmd : Inport
  VeSVMR_Pct_DC_DutyA_in : Inport  Port=2
  VeSVMR_Pct_DC_DutyB_in : Inport  Port=3
  VeSVMR_Pct_DC_DutyC_in : Inport  Port=4
  VeMCDR_I_IsdCmd : Inport  Port=5
  VeMCDR_I_IsqCmd : Inport  Port=6
  VeSVMC_r_CosPwm : Inport  Port=7
  VeSVMC_r_SinPwm : Inport  Port=8
  VaSVMR_K_DeadTimeCmp_Slope : Inport  Port=9
  VaSVMR_Pct_DeadTimeCmp : Inport  Port=10
  VeSVMR_e_PWM_Type : Inport  Port=11
  VeSVMR_Pct_DC_FixedDutyOffset : Inport  Port=12
  VaSVMR_Pct_DCMaxDuty_nom : Inport  Port=13
  VaSVMR_Pct_DCMinDuty_nom : Inport  Port=14
  VaSVMR_Pct_DCMaxDutyRound : Inport  Port=15
  VaSVMR_Pct_DCMinDutyRound : Inport  Port=16
  VeMCCR_b_UseMeasCrntDTC : Inport  Port=17
  LeMCCR_I_TmpIq : Inport  Port=18
  LeMCCR_I_TmpId : Inport  Port=19
  Comparison3 : RelationalOperator  Operator===  OutDataTypeStr=boolean  InputSameDT=off
  Constant14 : Constant
      settings: AttributesFormatString=dd_value = 1
  If : If  IfExpression=u1 ~= 0
  If Action Subsystem : Subsystem  TreatAsAtomicUnit=on
  If Action Subsystem1 : Subsystem  TreatAsAtomicUnit=on
  If Action Subsystem5 : Subsystem  TreatAsAtomicUnit=on
  If Action Subsystem6 : Subsystem  TreatAsAtomicUnit=on
  If2 : If  IfExpression=u1 ~= 0
  Logical Operator : Logic  Operator=OR  AllPortsSameDT=off  OutDataTypeStr=boolean
  Merge{,1..7} (8 alike) : Merge
  ReciSqrt3M1 : Constant  OutDataTypeStr=uint8
      settings: AttributesFormatString=dd_value = 1
  ReciSqrt3M2 : Constant  Value=0  OutDataTypeStr=uint8
      settings: AttributesFormatString=dd_value = 0
  Relational Operator : RelationalOperator  Operator===  OutDataTypeStr=boolean  InputSameDT=off
  Relational Operator1 : RelationalOperator  Operator===  OutDataTypeStr=boolean  InputSameDT=off
  Signal Conversion : SignalConversion  OverrideOpt=off
  VeSVMR_Pct_DC_DutyA_Cmd : Outport  VectorParamsAs1DForOutWhenUnconnected=off
  VeSVMR_Pct_DC_DutyB_Cmd : Outport  Port=2  VectorParamsAs1DForOutWhenUnconnected=off
  VeSVMR_Pct_DC_DutyC_Cmd : Outport  Port=3  VectorParamsAs1DForOutWhenUnconnected=off
  VeSVMR_Pct_DC_DutyA : Outport  Port=4  VectorParamsAs1DForOutWhenUnconnected=off
  VeSVMR_Pct_DC_DutyB : Outport  Port=5  VectorParamsAs1DForOutWhenUnconnected=off
  VeSVMR_Pct_DC_DutyC : Outport  Port=6  VectorParamsAs1DForOutWhenUnconnected=off
  wires:
  Merge2/1 -> VeSVMR_Pct_DC_DutyC/1
  Merge1/1 -> VeSVMR_Pct_DC_DutyB/1
  Merge/1 -> VeSVMR_Pct_DC_DutyA/1
  Merge6/1 -> VeSVMR_Pct_DC_DutyC_Cmd/1
  Merge5/1 -> VeSVMR_Pct_DC_DutyB_Cmd/1
  Merge4/1 -> VeSVMR_Pct_DC_DutyA_Cmd/1
  If Action Subsystem1/3(VeSVMR_Pct_DC_DutyC_Cmd) -> Merge6/2
  If Action Subsystem/3(VeSVMR_Pct_DC_DutyC_Cmd) -> Merge6/1
  If Action Subsystem1/2(VeSVMR_Pct_DC_DutyB_Cmd) -> Merge5/2
  If Action Subsystem/2(VeSVMR_Pct_DC_DutyB_Cmd) -> Merge5/1
  If Action Subsystem1/1(VeSVMR_Pct_DC_DutyA_Cmd) -> Merge4/2
  If Action Subsystem/1(VeSVMR_Pct_DC_DutyA_Cmd) -> Merge4/1
  If Action Subsystem1/6(LeSVMC_Pct_DC_DutyC) -> Merge2/2
  If Action Subsystem/6(LeSVMC_Pct_DC_DutyC) -> Merge2/1
  If Action Subsystem1/5(LeSVMC_Pct_DC_DutyB) -> Merge1/2
  If Action Subsystem/5(LeSVMC_Pct_DC_DutyB) -> Merge1/1
  If Action Subsystem1/4(LeSVMC_Pct_DC_DutyA) -> Merge/2
  If Action Subsystem/4(LeSVMC_Pct_DC_DutyA) -> Merge/1
  If/2 -> If Action Subsystem1/Action
  VaSVMR_Pct_DCMinDutyRound/1 -> If Action Subsystem/15(VaSVMR_Pct_DCMinDutyRound)
  VaSVMR_Pct_DCMaxDutyRound/1 -> If Action Subsystem/14(VaSVMR_Pct_DCMaxDutyRound)
  VaSVMR_Pct_DCMinDuty_nom/1 -> If Action Subsystem/13(VaSVMR_Pct_DCMinDuty_nom)
  VaSVMR_Pct_DCMaxDuty_nom/1 -> If Action Subsystem/12(VaSVMR_Pct_DCMaxDuty_nom)
  VeSVMR_Pct_DC_FixedDutyOffset/1 -> If Action Subsystem/11(VeSVMR_Pct_DC_FixedDutyOffset)
  VeSVMR_e_PWM_Type/1 -> If Action Subsystem/10(VeSVMR_e_PWM_Type)
  VaSVMR_Pct_DeadTimeCmp/1 -> If Action Subsystem/9(VaSVMR_Pct_DeadTimeCmp)
  VaSVMR_K_DeadTimeCmp_Slope/1 -> If Action Subsystem/8(VaSVMR_K_DeadTimeCmp_Slope)
  [VeSVMC_r_SinPwm] -> If Action Subsystem/7(VeSVMC_r_SinPwm)
  [VeSVMC_r_CosPwm] -> If Action Subsystem/6(VeSVMC_r_CosPwm)
  [VeMCCR_I_Iqx] -> If Action Subsystem/5(VeMCCR_I_Iqx)
  [VeMCCR_I_Idx] -> If Action Subsystem/4(VeMCCR_I_Idx)
  VeSVMC_r_SinPwm/1 -> [VeSVMC_r_SinPwm]
  VeSVMC_r_CosPwm/1 -> [VeSVMC_r_CosPwm]
  VeSVMR_Pct_DC_DutyC_in/1 -> If Action Subsystem/3(VeSVMR_Pct_DC_DutyC)
  VeSVMR_Pct_DC_DutyB_in/1 -> If Action Subsystem/2(VeSVMR_Pct_DC_DutyB)
  VeSVMR_Pct_DC_DutyA_in/1 -> If Action Subsystem/1(VeSVMR_Pct_DC_DutyA)
  If/1 -> If Action Subsystem/Action
  Logical Operator/1 -> If/1
  Relational Operator1/1 -> Logical Operator/2
  Relational Operator/1 -> Logical Operator/1
  ReciSqrt3M2/1 -> Relational Operator1/2
  [LeSVMR_e_PwrStageCmd] -> Relational Operator1/1
  ReciSqrt3M1/1 -> Relational Operator/2
  [LeSVMR_e_PwrStageCmd] -> Relational Operator/1
  Signal Conversion/1 -> [LeSVMR_e_PwrStageCmd]
  VeGDCR_e_EffectivePwrStageCmd/1 -> Signal Conversion/1
  VeMCCR_b_UseMeasCrntDTC/1 -> Comparison3/1
  Constant14/1 -> Comparison3/2
  Comparison3/1 -> If2/1
  If2/1 -> If Action Subsystem5/Action
  If2/2 -> If Action Subsystem6/Action
  If Action Subsystem5/1(VeMCCR_I_Iqx) -> Merge3/1
  Merge3/1 -> [VeMCCR_I_Iqx]  "VeMCCR_I_Iqx"
  If Action Subsystem5/2(VeMCCR_I_Idx) -> Merge7/1
  Merge7/1 -> [VeMCCR_I_Idx]  "VeMCCR_I_Idx"
  If Action Subsystem6/1(VeMCCR_I_Iqx) -> Merge3/2
  If Action Subsystem6/2(VeMCCR_I_Idx) -> Merge7/2
  LeMCCR_I_TmpIq/1 -> If Action Subsystem5/1(LeMCCR_I_TmpIq)
  LeMCCR_I_TmpId/1 -> If Action Subsystem5/2(LeMCCR_I_TmpId)
  VeMCDR_I_IsqCmd/1 -> If Action Subsystem6/1(VeMCDR_I_IsqCmd)
  VeMCDR_I_IsdCmd/1 -> If Action Subsystem6/2(VeMCDR_I_IsdCmd)

== system pdc_grc/PDC/PWMCalculation/DeadTimeCompensation/ReInitSVMR_DeadTimeCompensation ==
  Constant : Constant  Value=KeSVMR_t_DeadTime
      settings: AttributesFormatString=dd_value = 1.8e-06
  Constant2 : Constant  Value=KeSVMR_PWMPrd_cnt  OutDataTypeStr=single
  Constant3 : Constant  Value=KeSVMR_FullDTCCurr_A
      settings: AttributesFormatString=dd_value = 8
  Constant4 : Constant  Value=single(1)
      settings: AttributesFormatString=dd_value = 1
  Divide1 : Product  Inputs=*/
  Product : Product
  Product1 : Product
  Signal Conversion : SignalConversion  OverrideOpt=off
  Signal Conversion1 : SignalConversion  OverrideOpt=off
  VeSVMR_K_DeadTimeCmp_Slope : Outport  VectorParamsAs1DForOutWhenUnconnected=off
  VeSVMR_Pct_DeadTimeCmp : Outport  Port=2  VectorParamsAs1DForOutWhenUnconnected=off
  wires:
  Signal Conversion1/1 -> VeSVMR_Pct_DeadTimeCmp/1
  Signal Conversion/1 -> VeSVMR_K_DeadTimeCmp_Slope/1
  Product/1 -> Signal Conversion1/1, Product1/2
  Divide1/1 -> Product1/1
  Constant4/1 -> Divide1/1
  Constant3/1 -> Divide1/2
  Product1/1 -> Signal Conversion/1
  Constant2/1 -> Product/2
  Constant/1 -> Product/1

== system pdc_grc/PDC/PWMCalculation/DeadTimeCompensation/ReInitSVMR_PWM_Modulation ==
  Constant2 : Constant  Value=KeSVMR_PWMPrd_cnt  OutDataTypeStr=single
  Constant3 : Constant
      settings: AttributesFormatString=dd_value = 1
  Constant5 : Constant  Value=KeSVMR_b_UseStrictClamp
      settings: AttributesFormatString=dd_value = 0
  Constant6 : Constant
      settings: AttributesFormatString=dd_value = 1
  If : If  IfExpression=u1 ~= 0
  Logical Operator : Logic  AllPortsSameDT=off  OutDataTypeStr=boolean
  Merge : Merge
  Merge1 : Merge
  Merge2 : Merge
  Not_SVPWM_StrictClamp : Subsystem  TreatAsAtomicUnit=on
  ReciSqrt3M2 : Constant  OutDataTypeStr=uint8
      settings: AttributesFormatString=dd_value = 1
  Relational Operator1 : RelationalOperator  Operator===  OutDataTypeStr=boolean  InputSameDT=off
  Relational Operator2 : RelationalOperator  Operator===  OutDataTypeStr=boolean  InputSameDT=off
  SVPWM_StrictClamp : Subsystem  TreatAsAtomicUnit=on
  VeSVMR_Pct_DC_FixedDutyOffset : Outport  VectorParamsAs1DForOutWhenUnconnected=off
  VeSVMR_Pct_DCMaxDuty_nom : Outport  Port=2  VectorParamsAs1DForOutWhenUnconnected=off
  VeSVMR_Pct_DCMinDuty_nom : Outport  Port=3  VectorParamsAs1DForOutWhenUnconnected=off
  VeSVMR_Pct_DCMaxDutyRound : Outport  Port=4  VectorParamsAs1DForOutWhenUnconnected=off
  VeSVMR_Pct_DCMinDutyRound : Outport  Port=5  VectorParamsAs1DForOutWhenUnconnected=off
  wires:
  Merge2/1 -> VeSVMR_Pct_DC_FixedDutyOffset/1
  Not_SVPWM_StrictClamp/4(VeSVMR_Pct_DCMinDutyRound) -> VeSVMR_Pct_DCMinDutyRound/1
  Not_SVPWM_StrictClamp/3(VeSVMR_Pct_DCMaxDutyRound) -> VeSVMR_Pct_DCMaxDutyRound/1
  Merge1/1 -> VeSVMR_Pct_DCMaxDuty_nom/1
  Not_SVPWM_StrictClamp/5(VeSVMR_Pct_DC_FixedDutyOffset) -> Merge2/2
  SVPWM_StrictClamp/3(VeSVMR_Pct_DC_FixedDutyOffset) -> Merge2/1
  Not_SVPWM_StrictClamp/2(VeSVMR_Pct_DCMaxDuty_nom) -> Merge1/2
  SVPWM_StrictClamp/2(VaSVMR_Pct_DCMaxDuty_nom) -> Merge1/1
  Not_SVPWM_StrictClamp/1(VeSVMR_Pct_DCMinDuty_nom) -> Merge/2
  SVPWM_StrictClamp/1(VaSVMR_Pct_DCMinDuty_nom) -> Merge/1
  If/1 -> SVPWM_StrictClamp/Action
  If/2 -> Not_SVPWM_StrictClamp/Action
  Logical Operator/1 -> If/1
  Relational Operator1/1 -> Logical Operator/2
  Relational Operator2/1 -> Logical Operator/1
  Constant6/1 -> Relational Operator2/2
  Constant5/1 -> Relational Operator2/1
  Constant3/1 -> Relational Operator1/2
  Merge/1 -> VeSVMR_Pct_DCMinDuty_nom/1
  ReciSqrt3M2/1 -> Relational Operator1/1
  Constant2/1 -> Not_SVPWM_StrictClamp/1(LeSVMR_f_InvTs)

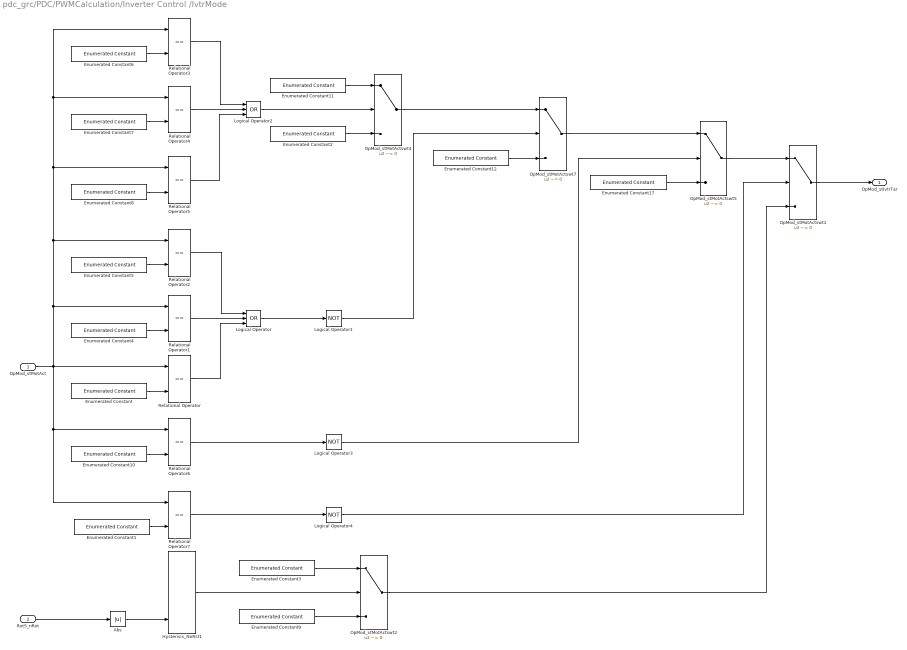
== system pdc_grc/PDC/PWMCalculation/Inverter Control /IvtrMode ==
  OpMod_stMotAct : Inport
  RotS_nRot : Inport  Port=2  OutDataTypeStr=single
  Abs : Abs  SaturateOnIntegerOverflow=off
  Enumerated Constant : simulink/Sources/Enumerated Constant  OutDataTypeStr=Enum: StMotMod  Value=StMotMod.StMotModTqCtrl  SampleTime=inf
  Enumerated Constant1 : simulink/Sources/Enumerated Constant  OutDataTypeStr=Enum: StMotMod  Value=StMotMod.StMotModFailure  SampleTime=inf
  Enumerated Constant10 : simulink/Sources/Enumerated Constant  OutDataTypeStr=Enum: StMotMod  Value=StMotMod.StMotModAfterRun  SampleTime=inf
  Enumerated Constant11 : simulink/Sources/Enumerated Constant  OutDataTypeStr=Enum: StIvtrMod  Value=StIvtrMod.StIvtrModFW  SampleTime=inf
  Enumerated Constant12 : simulink/Sources/Enumerated Constant  OutDataTypeStr=Enum: StIvtrMod  Value=StIvtrMod.StIvtrModDtcyCtrl  SampleTime=inf
  Enumerated Constant17 : simulink/Sources/Enumerated Constant  OutDataTypeStr=Enum: StIvtrMod  Value=StIvtrMod.StIvtrModIvtrOffMod  SampleTime=inf
  Enumerated Constant2 : simulink/Sources/Enumerated Constant  OutDataTypeStr=Enum: StIvtrMod  Value=StIvtrMod.StIvtrModFW  SampleTime=inf
  Enumerated Constant3 : simulink/Sources/Enumerated Constant  OutDataTypeStr=Enum: StIvtrMod  Value=StIvtrMod.StIvtrModASCLo  SampleTime=inf
  Enumerated Constant4 : simulink/Sources/Enumerated Constant  OutDataTypeStr=Enum: StMotMod  Value=StMotMod.StMotModDischarge  SampleTime=inf
  Enumerated Constant5 : simulink/Sources/Enumerated Constant  OutDataTypeStr=Enum: StMotMod  Value=StMotMod.StMotModSpdCtrl  SampleTime=inf
  Enumerated Constant6 : simulink/Sources/Enumerated Constant  OutDataTypeStr=Enum: StMotMod  Value=StMotMod.StMotModIni  SampleTime=inf
  Enumerated Constant7 : simulink/Sources/Enumerated Constant  OutDataTypeStr=Enum: StMotMod  Value=StMotMod.StMotModStandby  SampleTime=inf
  Enumerated Constant8 : simulink/Sources/Enumerated Constant  OutDataTypeStr=Enum: StMotMod  Value=StMotMod.StMotModReady  SampleTime=inf
  Enumerated Constant9 : simulink/Sources/Enumerated Constant  OutDataTypeStr=Enum: StIvtrMod  Value=StIvtrMod.StIvtrModFW  SampleTime=inf
  Hysterisis_NoRst1 : GRC_Lib/Nonlinear/Hysterisis_NoRst  SystemSampleTime=-1  VariantActivationTime=update diagram  AllowFlexibleInterface=on  Latency=0  AutoFrameSizeCalculation=off
  Logical Operator : Logic  Operator=OR  Inputs=3  AllPortsSameDT=off  OutDataTypeStr=boolean
  Logical Operator1 : Logic  Operator=NOT  AllPortsSameDT=off  OutDataTypeStr=boolean
  Logical Operator2 : Logic  Operator=OR  Inputs=3  AllPortsSameDT=off  OutDataTypeStr=boolean
  Logical Operator3 : Logic  Operator=NOT  AllPortsSameDT=off  OutDataTypeStr=boolean
  Logical Operator4 : Logic  Operator=NOT  AllPortsSameDT=off  OutDataTypeStr=boolean
  OpMod_stMotActswt{1..2,4..5,7} (5 alike) : Switch  Criteria=u2 ~= 0  SaturateOnIntegerOverflow=off  InputSameDT=off
  Relational Operator{,1..7} (8 alike) : RelationalOperator  Operator===  OutDataTypeStr=boolean  RndMeth=Simplest  InputSameDT=off
  OpMod_stIvtrTar : Outport  VectorParamsAs1DForOutWhenUnconnected=off
  wires:
  Relational Operator/1 -> Logical Operator/3
  Enumerated Constant/1 -> Relational Operator/2
  RotS_nRot/1 -> Abs/1
  Abs/1 -> Hysterisis_NoRst1/3
  Enumerated Constant4/1 -> Relational Operator1/2
  Relational Operator1/1 -> Logical Operator/2
  Enumerated Constant5/1 -> Relational Operator2/2
  Relational Operator2/1 -> Logical Operator/1
  Enumerated Constant6/1 -> Relational Operator3/2
  Enumerated Constant7/1 -> Relational Operator4/2
  Enumerated Constant8/1 -> Relational Operator5/2
  Relational Operator5/1 -> Logical Operator2/3
  Relational Operator4/1 -> Logical Operator2/2
  Relational Operator3/1 -> Logical Operator2/1
  Logical Operator2/1 -> OpMod_stMotActswt4/2
  Enumerated Constant2/1 -> OpMod_stMotActswt4/3
  Enumerated Constant10/1 -> Relational Operator6/2
  OpMod_stMotAct/1 -> Relational Operator7/1, Relational Operator6/1, Relational Operator/1, Relational Operator3/1, Relational Operator4/1, Relational Operator5/1, Relational Operator2/1, Relational Operator1/1
  Enumerated Constant12/1 -> OpMod_stMotActswt7/3
  Logical Operator/1 -> Logical Operator1/1
  OpMod_stMotActswt4/1 -> OpMod_stMotActswt7/1
  Relational Operator6/1 -> Logical Operator3/1
  OpMod_stMotActswt7/1 -> OpMod_stMotActswt5/1
  Enumerated Constant17/1 -> OpMod_stMotActswt5/3
  OpMod_stMotActswt5/1 -> OpMod_stMotActswt1/1
  OpMod_stMotActswt1/1 -> OpMod_stIvtrTar/1
  Enumerated Constant11/1 -> OpMod_stMotActswt4/1
  Enumerated Constant1/1 -> Relational Operator7/2
  Hysterisis_NoRst1/1 -> OpMod_stMotActswt2/2
  Relational Operator7/1 -> Logical Operator4/1
  Enumerated Constant3/1 -> OpMod_stMotActswt2/1
  Enumerated Constant9/1 -> OpMod_stMotActswt2/3
  OpMod_stMotActswt2/1 -> OpMod_stMotActswt1/3
  Logical Operator1/1 -> OpMod_stMotActswt7/2
  Logical Operator3/1 -> OpMod_stMotActswt5/2
  Logical Operator4/1 -> OpMod_stMotActswt1/2

== system pdc_grc/PDC/PWMCalculation/PWMCmdCtrlEnable/NormalPWM ==
  Normal_PWM_Duty : Inport
  Action Port : ActionPort
  Constant : Constant  OutDataTypeStr=uint8
  PWM_Duty : Outport  VectorParamsAs1DForOutWhenUnconnected=off
  PDC_Ivtr1ModCmd : Outport  Port=2  VectorParamsAs1DForOutWhenUnconnected=off
  wires:
  Normal_PWM_Duty/1 -> PWM_Duty/1
  Constant/1 -> PDC_Ivtr1ModCmd/1

== system pdc_grc/PDC/PWMCalculation/PWMCmdCtrlEnable/PWMFW ==
  Action Port : ActionPort
  0% : Constant  Value=0.5  OutDataTypeStr=single
  0%1 : Constant  Value=0.5  OutDataTypeStr=single
  0%2 : Constant  Value=0.5  OutDataTypeStr=single
  C Caller1 : CCaller  FunctionName=gatedriver_disable
  Constant : Constant  Value=0  OutDataTypeStr=uint8
  Mux : Mux  Inputs=3
  PWM_Duty : Outport  VectorParamsAs1DForOutWhenUnconnected=off
  PDC_Ivtr1ModCmd : Outport  Port=2  VectorParamsAs1DForOutWhenUnconnected=off
  wires:
  0%2/1 -> Mux/3
  0%1/1 -> Mux/2
  0%/1 -> Mux/1
  Mux/1 -> PWM_Duty/1
  Constant/1 -> PDC_Ivtr1ModCmd/1

== system pdc_grc/PDC/PWMCalculation/PWMCmdCtrlEnable/PWMGOFF ==
  PWMType : Inport
  Action Port : ActionPort
  0% : Constant  Value=0  OutDataTypeStr=single
  0%1 : Constant  Value=0  OutDataTypeStr=single
  0%2 : Constant  Value=0  OutDataTypeStr=single
  Mux : Mux  Inputs=3
  PWM_Duty : Outport  VectorParamsAs1DForOutWhenUnconnected=off
  PDC_Ivtr1ModCmd : Outport  Port=2  VectorParamsAs1DForOutWhenUnconnected=off
  wires:
  PWMType/1 -> PDC_Ivtr1ModCmd/1
  Mux/1 -> PWM_Duty/1
  0%/1 -> Mux/1
  0%1/1 -> Mux/2
  0%2/1 -> Mux/3

== system pdc_grc/PDC/PWMCalculation/PWMCmdCtrlEnable/ThreePhaseSC ==
  NormalPWMDuty : Inport
  PWMType : Inport  Port=2
  CCM_ASCEna : Inport  Port=3
  Action Port : ActionPort  InitializeStates=reset
  ASC2 : Stateflow chart  TreatAsAtomicUnit=on
  Constant2 : Constant  Value=KPDC_FWCnt_C
  PWM_Duty : Outport  VectorParamsAs1DForOutWhenUnconnected=off
  PDC_Ivtr1ModCmd : Outport  Port=2  OutDataTypeStr=uint8  VectorParamsAs1DForOutWhenUnconnected=off
  wires:
  Constant2/1 -> ASC2/3(fwCnt)
  PWMType/1 -> ASC2/1(PWMType)
  ASC2/1(PDC_Ivtr1ModCmd) -> PDC_Ivtr1ModCmd/1
  CCM_ASCEna/1 -> ASC2/2(ASCPWMEna)
  NormalPWMDuty/1 -> ASC2/4(Duty)
  ASC2/2(ActDuty) -> PWM_Duty/1

== system pdc_grc/PDC/PWMCalculation/PWMCmdCtrlEnable/ThreePhaseSC1 ==
  PWMType : Inport
  Action Port : ActionPort  InitializeStates=reset
  ASC : Stateflow chart  TreatAsAtomicUnit=on
  Constant1 : Constant  Value=KASC_DecDuty_value
  Constant2 : Constant  Value=KASC_OpenTime_s
  Constant3 : Constant  Value=KCCM_ASCSwitchEna_flg
  Mux : Mux  Inputs=3
  PWM_Duty : Outport  VectorParamsAs1DForOutWhenUnconnected=off
  PDC_Ivtr1ModCmd : Outport  Port=2  OutDataTypeStr=uint8  VectorParamsAs1DForOutWhenUnconnected=off
  wires:
  ASC/4(PDC_Ivtr1ModCmd) -> PDC_Ivtr1ModCmd/1
  PWMType/1 -> ASC/4(PWMType)
  ASC/3(ActDutyW) -> Mux/3
  ASC/2(ActDutyV) -> Mux/2
  ASC/1(ActDutyU) -> Mux/1
  Constant2/1 -> ASC/3(OpenTime_s)
  Constant1/1 -> ASC/2(Duty)
  Constant3/1 -> ASC/1(KCCM_ASCSwitchEna_flg)
  Mux/1 -> PWM_Duty/1
